simulink model "analog_tp_2"  (Simulink 7.7)
settings: Solver=ode45  StartTime=0.0  StopTime=0.5  MaxStep=dt  RelTol=1e-3
values from neighbouring files (symbols this model uses):
  a = zeros(5, nord+1)    [analog_tp1.m]    (also in analog_tp2.m)
  b = fir1(nr-1,0.5)    [adapt_filter1.m]    (also in adapt_filter2.m; analog_tp1.m = zeros(5, nord+1); analog_tp2.m = zeros(5, nord+1))
  delay = verz(Typ)    [analog_hp11.m]    (also in analog_hp12.m; analog_tp11.m; analog_tp12.m; analog_tp2.m = 0.001)
  f1 = 0.1    [CFIR_1.m]    (also in analog_bp1.m = ',num2str(f1),' Hz; analog_bp11.m = ',num2str(f1),' Hz; analog_bp2.m = 30000; analog_bp3.m = 30000)
  f2 = 0.3    [CFIR_1.m]    (also in analog_bp1.m = ',num2str(f2),' Hz)']); analog_bp11.m = ',num2str(f2),' Hz)']); analog_bp2.m = 35000; analog_bp3.m = 30500)
  f3 = 500    [analog_tp2.m]
  frausch = 250    [analog_bp3.m]    (also in analog_tp2.m = 500)
  frechteck = 20    [analog_tp2.m]
  K1 = 0    [analog_tp2.m]
  K2 = 0    [analog_tp2.m]
  K3 = 0    [analog_tp2.m]
  Kdreieck = 0    [analog_tp2.m]
  Krausch = 1    [analog_tp2.m]
  Krechteck = 0    [analog_tp2.m]
  Typ = 2    [analog_bp1.m]    (also in analog_bp2.m = 4; analog_bp3.m; analog_tp13.m; analog_tp2.m)
libraries: dsparch4 x1
settings Model: Creator=svenhoffmann  LastModifiedBy=josef  ExtModeAutoUpdateStatusClock=off
settings DataIOCC: MaxDataPoints=2000  SignalLoggingName=sigsOut
settings DebuggingCC: SaveWithParameterizedLinksMsg=none  SignalResolutionControl=TryResolveAllWithWarning  SolverPrmCheckMsg=none  MultiTaskDSMMsg=warning  MultiTaskCondExecSysMsg=none  StrictBusMsg=None
settings HardwareCC: TargetUnknown=on
settings RTWCC: IncludeERTFirstTime=on

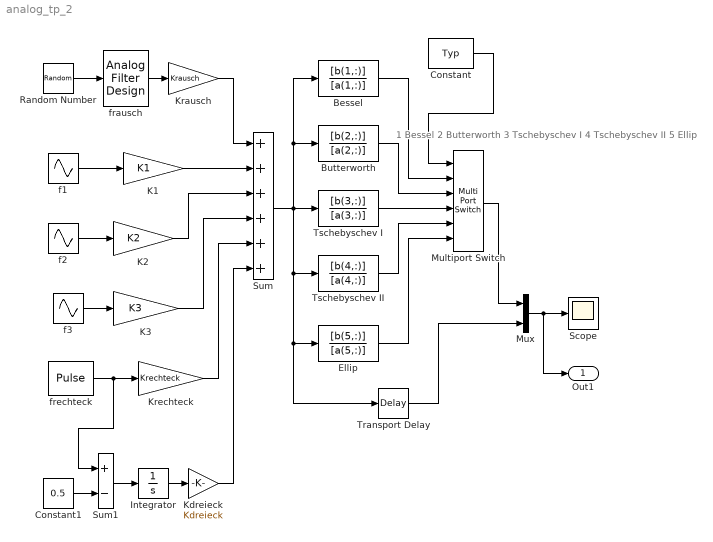
== system analog_tp_2 ==
  note: 1 Bessel
      | 2 Butterworth
      | 3 Tschebyschev I
      | 4 Tschebyschev II
      | 5 Ellip
  Bessel : TransferFcn  Numerator=[b(1,:)]  Denominator=[a(1,:)]
  Butterworth : TransferFcn  Numerator=[b(2,:)]  Denominator=[a(2,:)]
  Constant : Constant  Value=Typ
  Constant1 : Constant  Value=0.5
  Ellip : TransferFcn  Numerator=[b(5,:)]  Denominator=[a(5,:)]
  Integrator : Integrator
  K1 : Gain  Gain=K1  SaturateOnIntegerOverflow=on  OutDataTypeStr=Inherit: Same as input  ParamDataTypeStr=Inherit: Same as input
  K2 : Gain  Gain=K2  SaturateOnIntegerOverflow=on  OutDataTypeStr=Inherit: Same as input  ParamDataTypeStr=Inherit: Same as input
  K3 : Gain  Gain=K3  SaturateOnIntegerOverflow=on  OutDataTypeStr=Inherit: Same as input  ParamDataTypeStr=Inherit: Same as input
  Kdreieck : Gain  Gain=Kdreieck  SaturateOnIntegerOverflow=on  OutDataTypeStr=Inherit: Same as input  ParamDataTypeStr=Inherit: Same as input
  Krausch : Gain  Gain=Krausch  SaturateOnIntegerOverflow=on  OutDataTypeStr=Inherit: Same as input  ParamDataTypeStr=Inherit: Same as input
  Krechteck : Gain  Gain=Krechteck  SaturateOnIntegerOverflow=on  OutDataTypeStr=Inherit: Same as input  ParamDataTypeStr=Inherit: Same as input
  Multiport Switch : MultiPortSwitch  Inputs=5  zeroidx=off  InputSameDT=on
  Mux : Mux  Inputs=2
  Random Number : RandomNumber  SampleTime=0
  Scope : Scope
      settings: YMin=0  YMax=17.5
  Sum : Sum  Inputs=++++++  SaturateOnIntegerOverflow=on  InputSameDT=on  OutDataTypeStr=Inherit: Same as first input
  Sum1 : Sum  Inputs=+-  SaturateOnIntegerOverflow=on  InputSameDT=on  OutDataTypeStr=Inherit: Same as first input
  Transport Delay : TransportDelay  DelayTime=delay
  Tschebyschev I : TransferFcn  Numerator=[b(3,:)]  Denominator=[a(3,:)]
  Tschebyschev II : TransferFcn  Numerator=[b(4,:)]  Denominator=[a(4,:)]
  f1 : Sin  Frequency=2*pi*f1  SampleTime=0
  f2 : Sin  Amplitude=1/3  Frequency=2*pi*f2  SampleTime=0
  f3 : Sin  Amplitude=1/5  Frequency=2*pi*f3  SampleTime=0
  frausch : dsparch4/Analog Filter Design  method=Elliptic  filttype=Lowpass  N=8  Wlo=2*pi*frausch  Whi=80  Rp=0.1  Rs=60
  frechteck : DiscretePulseGenerator  PulseType=Time based  Period=1/frechteck  PulseWidth=50
  Out1 : Outport
  wires:
  Random Number/1 -> frausch/1
  f1/1 -> K1/1
  f2/1 -> K2/1
  f3/1 -> K3/1
  Krausch/1 -> Sum/1
  K1/1 -> Sum/2
  K2/1 -> Sum/3
  K3/1 -> Sum/4
  Sum/1 -> Butterworth/1, Bessel/1, Tschebyschev I/1, Tschebyschev II/1, Ellip/1, Transport Delay/1
  Bessel/1 -> Multiport Switch/2
  Butterworth/1 -> Multiport Switch/3
  Tschebyschev I/1 -> Multiport Switch/4
  Tschebyschev II/1 -> Multiport Switch/5
  Ellip/1 -> Multiport Switch/6
  Constant/1 -> Multiport Switch/1
  Mux/1 -> Scope/1, Out1/1
  Multiport Switch/1 -> Mux/1
  Transport Delay/1 -> Mux/2
  frausch/1 -> Krausch/1
  frechteck/1 -> Krechteck/1, Sum1/1
  Integrator/1 -> Kdreieck/1
  Sum1/1 -> Integrator/1
  Constant1/1 -> Sum1/2
  Krechteck/1 -> Sum/5
  Kdreieck/1 -> Sum/6
